simulink model "testAllanVar"  (R2018a)
settings: Solver=FixedStepDiscrete  StartTime=0.0  StopTime=inf  FixedStep=1/Fs  RelTol=1e-3
PreLoadFcn:
  | modelDef = getModelDef();
  | load VINS_bus_definitions.mat;
  | 
  | Fs = 1125;  % nominal IMU sampling rate (Hz)
  | 
  | gyroCalBiases = [0;0;0];
  | gyroCalMatrix = eye(3);
  | gyroGsensMatrix = zeros(3,3);
  | 
  | accelCalBiases = [0;0;0];
  | accelCalMatrix = eye(3);
  | 
  | imuPar = getImuPar('lmvpUncalibrated');
  | 
  | lastUsedMgyr = zeros(3,3);
  | 
  | simData = true;
libraries: dspsrcs4 x5, dspmtrx3 x2, dspswit3 x1, simulink x1
settings Model: Creator=Eric  LastModifiedBy=efoxlin
settings OptimizationCC: DefaultParameterBehavior=Inlined  UseFloatMulNetSlope=on  DefaultUnderspecifiedDataType=single  UseSpecifiedMinMax=on  InlineInvariantSignals=on  PassReuseOutputArgsAs=Individual arguments  NoFixptDivByZeroProtection=on  EfficientFloat2IntCast=on  LifeSpan=1  OptimizeBlockOrder=speed  DifferentSizesBufferReuse=on
settings DebuggingCC: ParameterTunabilityLossMsg=error  UnconnectedOutputMsg=none
settings HardwareCC: ProdBitPerPointer=32  ProdBitPerSizeT=32  ProdBitPerPtrDiffT=32  ProdLargestAtomicInteger=Long  ProdLargestAtomicFloat=Double  ProdWordSize=32  ProdHWDeviceType=ARM Compatible->ARM Cortex
settings SFSimCC: SimParseCustomCode=off  MATLABDynamicMemAlloc=off
settings RTWCC: SystemTargetFile=ert.tlc  GenCodeOnly=on  TemplateMakefile=ert_default_tmf  GenerateReport=on  Toolchain=Microsoft Visual C++ 2017 v15.0 | nmake (64-bit Windows)  BuildConfiguration=Faster Runs  IncludeHyperlinkInReport=on  LaunchReport=on  PortableWordSizes=on  TargetLang=C++  GenerateTraceInfo=on  GenerateTraceReport=on  GenerateTraceReportSl=on  GenerateTraceReportSf=on  GenerateTraceReportEml=on
settings CodeAppCC: ForceParamTrailComments=on  IgnoreCustomStorageClasses=off  OperatorAnnotations=on  SimulinkDataObjDesc=on  SFDataObjDesc=on  InsertBlockDesc=on
settings ERTTargetCC: TargetLangStandard=C++03 (ISO)  GenerateSampleERTMain=on  CombineSignalStateStructs=on  SuppressErrorStatus=on  SupportAbsoluteTime=off  MultiInstanceERTCode=on  CodeInterfacePackaging=C++ class  SupportNonFinite=off  SupportComplex=off  InlinedParameterPlacement=NonHierarchical  RootIOFormat=Structure reference  ERTCustomFileTemplate=example_file_process.tlc  ERTFilePackagingFormat=Compact

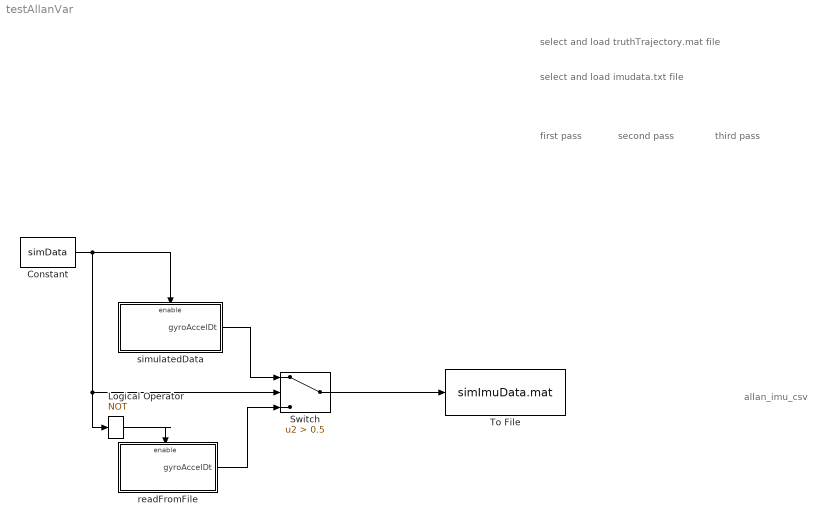
== system testAllanVar ==
  note: allan_imu_csv
  note: select and load imudata.txt file
  note: second pass
  note: first pass
  note: third pass
  note: select and load truthTrajectory.mat file
  Constant : Constant  Value=simData
  Logical Operator : Logic  Operator=NOT  IconShape=distinctive  AllPortsSameDT=off  OutDataTypeStr=boolean
  Switch : Switch  Criteria=u2 > Threshold  Threshold=0.5
  To File : ToFile  Filename=simImuData.mat  MatrixName=simImuData
  readFromFile : Subsystem
  simulatedData : Subsystem
  wires:
  readFromFile/1(gyroAccelDt) -> Switch/3
  simulatedData/1("gyroAccelDt ") -> Switch/1
  Constant/1 -> Logical Operator/1, Switch/2, simulatedData/Enable
  Logical Operator/1 -> readFromFile/Enable
  Switch/1 -> To File/1

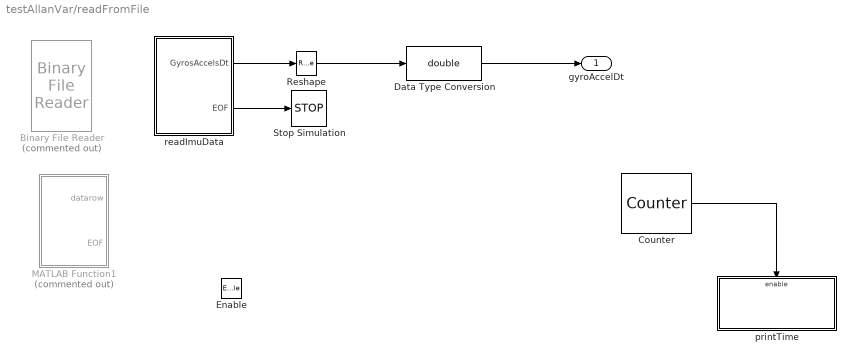
== system testAllanVar/readFromFile ==
  Enable : EnablePort
  Binary File Reader : dspsrcs4/Binary File Reader  Commented=on  Filename=GyroAccelDtFloat32.bin  HeaderStructure=struct([])  DataType=single  SamplesPerFrame=1  IsDataComplex=off  NumChannels=7  OutputEOF=on  SampleTime=1/Fs  SimulateUsing=Code generation
      settings: SourceProductName=DSP System Toolbox  SourceProductBaseCode=DS
  Counter : dspswit3/Counter  Direction=Up  CountEvent=Free running  CounterSize=User defined  MaxCount=4095  InitialCount=0  Output=Hit  HitValue=32  ResetInput=off  SamplesPerFrame=1  Ts=1/Fs  CntDtype=double  HitDtype=Logical
  Data Type Conversion : DataTypeConversion  OutDataTypeStr=double
  MATLAB Function1 : MATLAB Function  Commented=on  TreatAsAtomicUnit=on
  Reshape : Reshape  OutputDimensionality=Column vector (2-D)
  Stop Simulation : Stop
  printTime : Subsystem
  readImuData : Subsystem
  gyroAccelDt : Outport
  wires:
  Reshape/1 -> Data Type Conversion/1
  readImuData/1(GyrosAccelsDt) -> Reshape/1
  readImuData/2(EOF) -> Stop Simulation/1
  Data Type Conversion/1 -> gyroAccelDt/1
  Counter/1 -> printTime/Enable

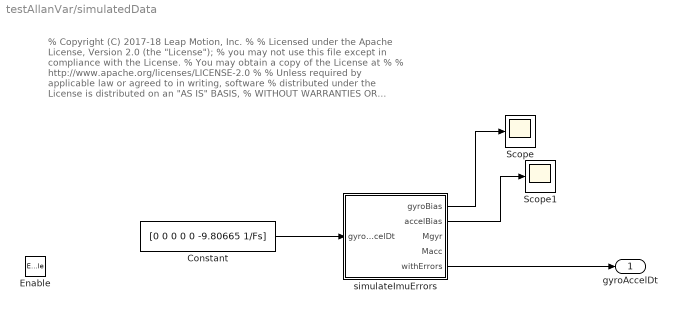
== system testAllanVar/simulatedData ==
  note: % Copyright (C) 2017-18 Leap Motion, Inc.
      | %
      | %    Licensed under the Apache License, Version 2.0 (the "License");
      | %    you may not use this file except in compliance with the License.
      | %    You may obtain a copy of the License at
      | %
      | %        http://www.apache.org/licenses/LICENSE-2.0
      | %
      | %    Unless required by applicable law or agreed to in writing, software
      | %    distributed under the License is distributed on an "AS IS" BASIS,
      | %    WITHOUT WARRANTIES OR CONDITIONS OF ANY KIND, either express or implied.
      | %    See the License for the specific language governing permissions and
      | %    limitations under the License.
      | % Author: Eric Foxlin
  Enable : EnablePort
  Constant : Constant  Value=[0 0 0 0 0 -9.80665 1/Fs]  SampleTime=1/Fs
  Scope : Scope
  Scope1 : Scope
  simulateImuErrors : Subsystem  TreatAsAtomicUnit=on
  "gyroAccelDt " : Outport
  wires:
  Constant/1 -> simulateImuErrors/1(gyroAccelDt)
  simulateImuErrors/5(withErrors) -> "gyroAccelDt "/1
  simulateImuErrors/1(gyroBias) -> Scope/1
  simulateImuErrors/2(accelBias) -> Scope1/1

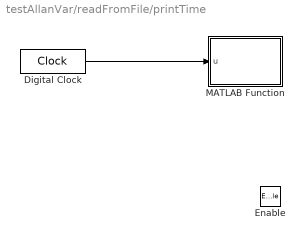
== system testAllanVar/readFromFile/printTime ==
  Enable : EnablePort
  Digital Clock : DigitalClock  SampleTime=1/Fs
  MATLAB Function : MATLAB Function  TreatAsAtomicUnit=on
  wires:
  Digital Clock/1 -> MATLAB Function/1(u)

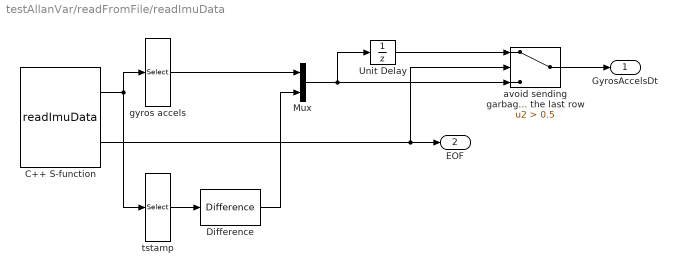
== system testAllanVar/readFromFile/readImuData ==
  C++ S-function : S-Function  FunctionName=readImuData  Parameters=1/Fs  SFunctionDeploymentMode=off  EnableBusSupport=off
  Difference : simulink/Discrete/Difference  ICPrevInput=0.0  OutMin=[]  OutMax=[]  OutDataType=fixdt(1, 16)  OutScaling=2^-10  DoSatur=off
  Mux : Mux  Inputs=2
  Unit Delay : UnitDelay  SampleTime=-1
  avoid sending garbage on the last row : Switch  Criteria=u2 > Threshold  Threshold=0.5
  gyros accels : Selector  InputPortWidth=10  IndexOptions=Index vector (dialog)  Indices=[4:9]  OutputSizes=1
  tstamp : Selector  InputPortWidth=10  IndexOptions=Index vector (dialog)  Indices=3  OutputSizes=1
  GyrosAccelsDt : Outport
  EOF : Outport  Port=2
  wires:
  C++ S-function/2 -> avoid sending garbage on the last row/2, EOF/1
  tstamp/1 -> Difference/1
  C++ S-function/1 -> gyros accels/1, tstamp/1
  gyros accels/1 -> Mux/1
  Mux/1 -> Unit Delay/1, avoid sending garbage on the last row/3
  Difference/1 -> Mux/2
  avoid sending garbage on the last row/1 -> GyrosAccelsDt/1
  Unit Delay/1 -> avoid sending garbage on the last row/1

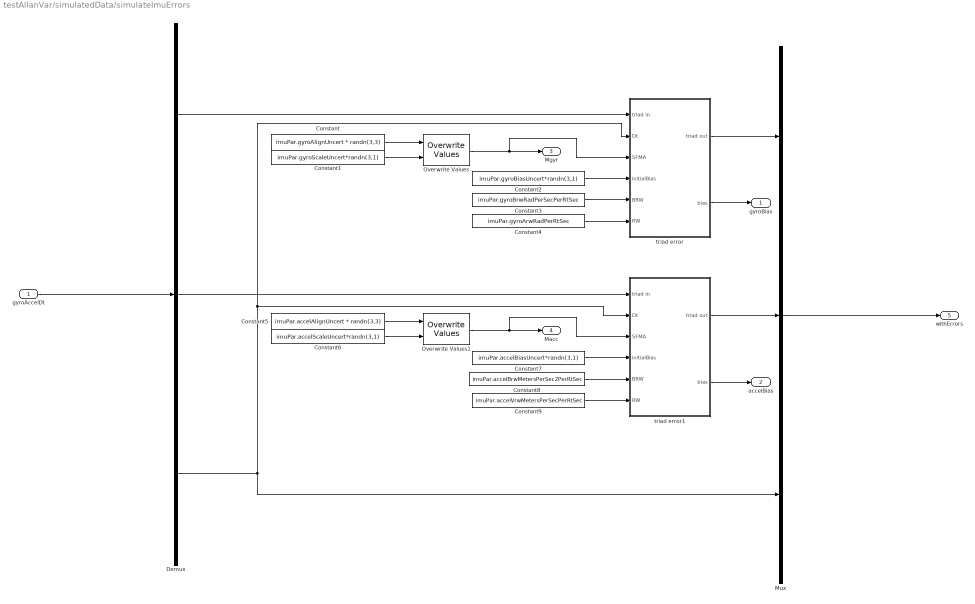
== system testAllanVar/simulatedData/simulateImuErrors ==
  gyroAccelDt : Inport
  Constant : Constant  Value=imuPar.gyroAlignUncert * randn(3,3)
  Constant1 : Constant  Value=imuPar.gyroScaleUncert*randn(3,1)
  Constant2 : Constant  Value=imuPar.gyroBiasUncert*randn(3,1)  VectorParams1D=off
  Constant3 : Constant  Value=imuPar.gyroBrwRadPerSecPerRtSec
  Constant4 : Constant  Value=imuPar.gyroArwRadPerRtSec
  Constant5 : Constant  Value=imuPar.accelAlignUncert * randn(3,3)
  Constant6 : Constant  Value=imuPar.accelScaleUncert*randn(3,1)
  Constant7 : Constant  Value=imuPar.accelBiasUncert*randn(3,1)  VectorParams1D=off
  Constant8 : Constant  Value=imuPar.accelBrwMetersPerSec2PerRtSec
  Constant9 : Constant  Value=imuPar.accelVrwMetersPerSecPerRtSec
  Demux : Demux  Outputs=[3 3 1]
  Mux : Mux  Inputs=3
  Overwrite Values : dspmtrx3/Overwrite Values  OverWriteDiag=Diagonal  valFrom2ndIP=Second input port  ConstValue=0  RowSpan=Range of rows  RowStartMode=First  RowStartIndex=1  RowEndMode=Last  RowEndIndex=1  ColSpan=Range of columns  ColStartMode=First  ColStartIndex=1  ColEndMode=Last  ColEndIndex=1  DiagSpan=All elements  DiagStartMode=Index  DiagStartIndex=2  DiagEndMode=Index  DiagEndIndex=4
      settings: SourceProductName=DSP System Toolbox  SourceProductBaseCode=DS
  Overwrite Values1 : dspmtrx3/Overwrite Values  OverWriteDiag=Diagonal  valFrom2ndIP=Second input port  ConstValue=0  RowSpan=Range of rows  RowStartMode=First  RowStartIndex=1  RowEndMode=Last  RowEndIndex=1  ColSpan=Range of columns  ColStartMode=First  ColStartIndex=1  ColEndMode=Last  ColEndIndex=1  DiagSpan=All elements  DiagStartMode=Index  DiagStartIndex=2  DiagEndMode=Index  DiagEndIndex=4
      settings: SourceProductName=DSP System Toolbox  SourceProductBaseCode=DS
  triad error : Subsystem  TreatAsAtomicUnit=on
  triad error1 : Subsystem  TreatAsAtomicUnit=on
  gyroBias : Outport
  accelBias : Outport  Port=2
  Mgyr : Outport  Port=3
  Macc : Outport  Port=4
  withErrors : Outport  Port=5
  wires:
  gyroAccelDt/1 -> Demux/1
  Demux/1 -> triad error/1(triad in)
  Demux/3 -> triad error1/2(Dt), triad error/2(Dt), Mux/3
  triad error/1(triad out) -> Mux/1
  Mux/1 -> withErrors/1
  Constant/1 -> Overwrite Values/1
  Constant1/1 -> Overwrite Values/2
  Overwrite Values/1 -> Mgyr/1, triad error/3(SFMA)
  Constant2/1 -> triad error/4(initialBias)
  triad error/2(bias) -> gyroBias/1
  Constant3/1 -> triad error/5(BRW)
  Constant4/1 -> triad error/6(RW)
  Constant7/1 -> triad error1/4(initialBias)
  Constant9/1 -> triad error1/6(RW)
  Constant8/1 -> triad error1/5(BRW)
  Constant6/1 -> Overwrite Values1/2
  Overwrite Values1/1 -> Macc/1, triad error1/3(SFMA)
  Constant5/1 -> Overwrite Values1/1
  Demux/2 -> triad error1/1(triad in)
  triad error1/1(triad out) -> Mux/2
  triad error1/2(bias) -> accelBias/1

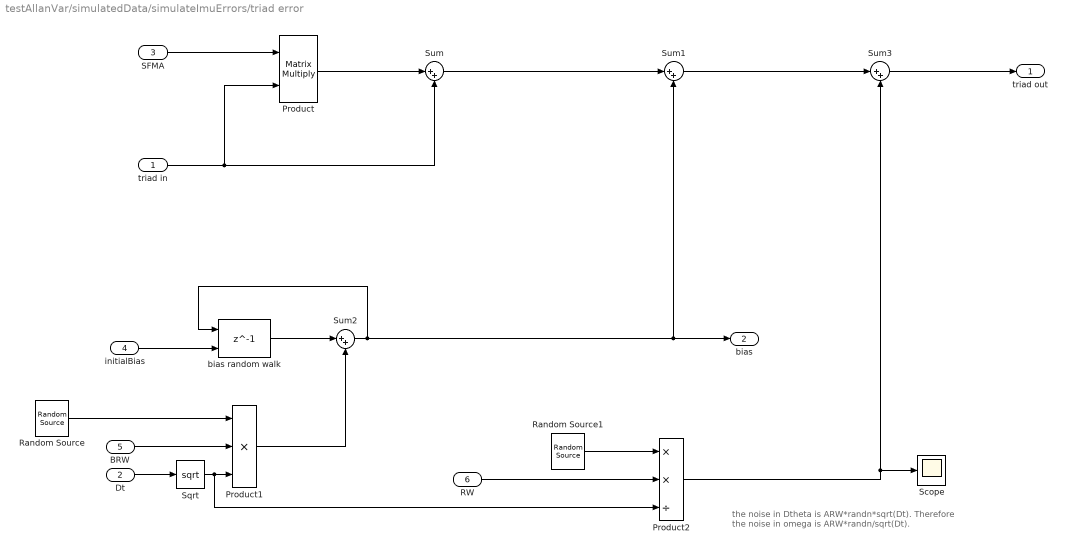
== system testAllanVar/simulatedData/simulateImuErrors/triad error ==
  note: the noise in Dtheta is ARW*randn*sqrt(Dt). Therefore the noise in omega is ARW*randn/sqrt(Dt).
  triad in : Inport
  Dt : Inport  Port=2
  SFMA : Inport  Port=3
  initialBias : Inport  Port=4
  BRW : Inport  Port=5
  RW : Inport  Port=6
  Product : Product  Multiplication=Matrix(*)
  Product1 : Product  Inputs=3
  Product2 : Product  Inputs=**/
  Random Source : dspsrcs4/Random Source  SrcType=Gaussian  NormMethod=Ziggurat  CltLength=12  MinVal=0  MaxVal=1  MeanVal=[0;0;0]  VarVal=1  RepMode=Not repeatable  rawSeed=1  IsInherit=off  SampMode=Discrete  SampTime=1/Fs  SampFrame=1  DataType=Double  OutComplex=Real  OutputFrames=off
  Random Source1 : dspsrcs4/Random Source  SrcType=Gaussian  NormMethod=Ziggurat  CltLength=12  MinVal=0  MaxVal=1  MeanVal=[0;0;0]  VarVal=1  RepMode=Not repeatable  rawSeed=1  IsInherit=off  SampMode=Discrete  SampTime=-1  SampFrame=1  DataType=Double  OutComplex=Real  OutputFrames=off
  Scope : Scope
  Sqrt : Sqrt  SaturateOnIntegerOverflow=on
  Sum{,1..3} (4 alike) : Sum  Inputs=|++
  bias random walk : Delay  DelayLength=1  InitialConditionSource=Input port
      settings: InputPortMap=u0,p4
  triad out : Outport
  bias : Outport  Port=2
  wires:
  triad in/1 -> Sum/2, Product/2
  SFMA/1 -> Product/1
  Product/1 -> Sum/1
  Sum/1 -> Sum1/1
  Sum1/1 -> Sum3/1
  initialBias/1 -> bias random walk/2
  bias random walk/1 -> Sum2/1
  Sum2/1 -> bias/1, Sum1/2, bias random walk/1
  Dt/1 -> Sqrt/1
  Sqrt/1 -> Product2/3, Product1/3
  BRW/1 -> Product1/2
  Product1/1 -> Sum2/2
  RW/1 -> Product2/2
  Sum3/1 -> triad out/1
  Product2/1 -> Scope/1, Sum3/2
  Random Source/1 -> Product1/1
  Random Source1/1 -> Product2/1

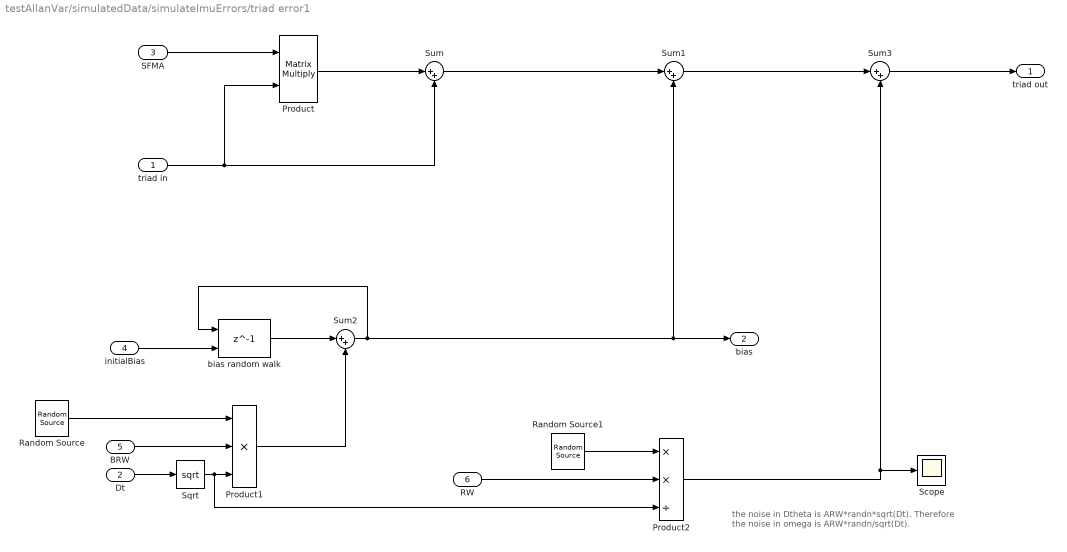
== system testAllanVar/simulatedData/simulateImuErrors/triad error1 ==
  note: the noise in Dtheta is ARW*randn*sqrt(Dt). Therefore the noise in omega is ARW*randn/sqrt(Dt).
  triad in : Inport
  Dt : Inport  Port=2
  SFMA : Inport  Port=3
  initialBias : Inport  Port=4
  BRW : Inport  Port=5
  RW : Inport  Port=6
  Product : Product  Multiplication=Matrix(*)
  Product1 : Product  Inputs=3
  Product2 : Product  Inputs=**/
  Random Source : dspsrcs4/Random Source  SrcType=Gaussian  NormMethod=Ziggurat  CltLength=12  MinVal=0  MaxVal=1  MeanVal=[0;0;0]  VarVal=1  RepMode=Not repeatable  rawSeed=1  IsInherit=off  SampMode=Discrete  SampTime=1/Fs  SampFrame=1  DataType=Double  OutComplex=Real  OutputFrames=off
  Random Source1 : dspsrcs4/Random Source  SrcType=Gaussian  NormMethod=Ziggurat  CltLength=12  MinVal=0  MaxVal=1  MeanVal=[0;0;0]  VarVal=1  RepMode=Not repeatable  rawSeed=1  IsInherit=off  SampMode=Discrete  SampTime=-1  SampFrame=1  DataType=Double  OutComplex=Real  OutputFrames=off
  Scope : Scope
  Sqrt : Sqrt  SaturateOnIntegerOverflow=on
  Sum{,1..3} (4 alike) : Sum  Inputs=|++
  bias random walk : Delay  DelayLength=1  InitialConditionSource=Input port
      settings: InputPortMap=u0,p4
  triad out : Outport
  bias : Outport  Port=2
  wires:
  triad in/1 -> Sum/2, Product/2
  SFMA/1 -> Product/1
  Product/1 -> Sum/1
  Sum/1 -> Sum1/1
  Sum1/1 -> Sum3/1
  initialBias/1 -> bias random walk/2
  bias random walk/1 -> Sum2/1
  Sum2/1 -> bias/1, Sum1/2, bias random walk/1
  Dt/1 -> Sqrt/1
  Sqrt/1 -> Product2/3, Product1/3
  BRW/1 -> Product1/2
  Product1/1 -> Sum2/2
  RW/1 -> Product2/2
  Sum3/1 -> triad out/1
  Product2/1 -> Scope/1, Sum3/2
  Random Source/1 -> Product1/1
  Random Source1/1 -> Product2/1

== matlab function testAllanVar/readFromFile/printTime/MATLAB Function ==
  data: u input
function  printTime(u)
%#codegen

% using fileId = 1  only generates a printf in the generated code
% fileId = 2 also causes prints in the matlab console

fprintf(1, "\r %f", u);

== matlab function testAllanVar/readFromFile/MATLAB Function1 ==
  data: datarow output; EOF output
function [datarow, EOF] = readLineAscii()

persistent data data2 nrows row

if isempty(data)
    % row format = # SeqID, DeviceID, timestamp (sec), gyroXYZ (rad/sec), accelXYZ (m/s^2), temperature (degC)
    coder.varsize('data', [500000, 10], [1 0]);  % ten columns,  up to 200k rows
    data = load('imudata.txt', '-ascii'); 
    
    validTimestamp = data(:,3) > 0.001;
    data2 = data(validTimestamp, [4 5 6 7 8 9 3]); % select just the useful columns and rows
    nrows = size(data2, 1);
    row = 2;  % skip the first row since we need delta-t's

end

datarow = data2(row,:)';
datarow(7) = data2(row,7) - data2(row-1,7); % calculate Delta-t

EOF = row >= nrows;
row = row + 1;
